simulink model "lab_readyAWU"  (R2020b)
settings: Solver=ode4  StartTime=0.0  StopTime=5  FixedStep=0.001  RelTol=1e-3
values from neighbouring files (symbols this model uses):
  degs2rpm = 0.166666666667    [DIGIT1-BE10.mat]    (also in DIGIT1-FE10.mat; DIGIT1-FE20.mat; DIGIT1-FE4.mat; DIGIT1-TR10.mat)
  filt =     [DIGIT1-BE10.mat]    (also in DIGIT1-FE10.mat; DIGIT1-FE20.mat; DIGIT1-FE4.mat; DIGIT1-TR10.mat)
  rpm2rads = 0.10471975512    [DIGIT1-BE10.mat]    (also in DIGIT1-FE10.mat; DIGIT1-FE20.mat; DIGIT1-FE4.mat; DIGIT1-TR10.mat)
  sens =     [DIGIT1-BE10.mat]    (also in DIGIT1-FE10.mat; DIGIT1-FE20.mat; DIGIT1-FE4.mat; DIGIT1-TR10.mat)
undefined symbols (not defined in the file or in its folder): National_Instruments, PCI
libraries: sldrtlib x3, simulink x1
settings Model: ExtModeTrigDuration=50001  Creator=verrimarco  LastModifiedBy=verrimarco
settings DataIOCC: SaveFormat=StructureWithTime  InspectSignalLogs=on  ReturnWorkspaceOutputs=off  LoggingFileName=out.mat2
settings RTWCC: Description=Simulink Desktop Real-Time  SystemTargetFile=sldrt.tlc  TemplateMakefile=sldrt.tmf  RTWCompilerOptimization=on
settings CodeAppCC: MaxIdLength=95
settings SimulinkDesktopRealTimeCC: TargetPreCompLibLocation=C:\Program Files\MATLAB\R2020b\toolbox\sldrt\lib\win64

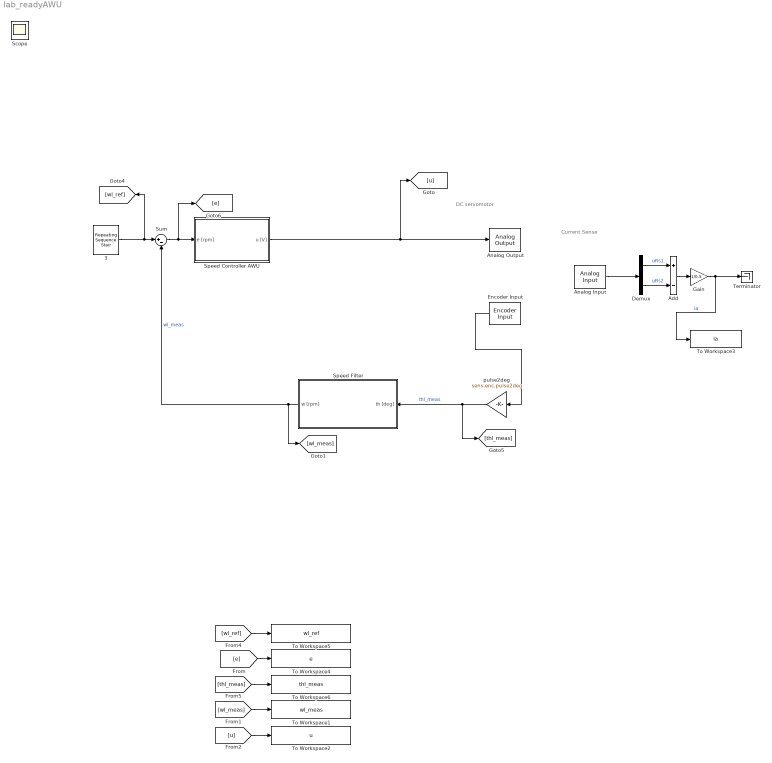
== system lab_readyAWU ==
  note: DC servomotor
  note: Current Sense
  3 : simulink/Sources/Repeating Sequence Stair  OutValues=[450 -450].'  tsamp=3  OutMin=[]  OutMax=[]  OutDataTypeStr=double  OutputDataTypeScalingMode=double  OutDataType=fixdt(0,8)  ConRadixGroup=Best Precision: Vector-wise  OutScaling=2^-12
  Add : Sum  Inputs=+-
  Analog Input : sldrtlib/Analog Input  SampleTime=-1  MaxMissedTicks=10  ShowMissedTicks=off  YieldWhenWaiting=off  DrvName=National_Instruments/PCI-6221  DrvAddress=4294967295  DrvOptions=[0 0 0 2 0]  Channels=[1,2]  RangeMode=1  VoltRange=1  DataType=1
      settings: AttributesFormatString=National Instruments\nPCI-6221 [auto]
  Analog Output : sldrtlib/Analog Output  SampleTime=-1  MaxMissedTicks=10  ShowMissedTicks=off  YieldWhenWaiting=off  DrvName=National_Instruments/PCI-6221  DrvAddress=4294967295  DrvOptions=[0 0 0 2 0]  Channels=1  RangeMode=1  VoltRange=1  InitialValue=0  FinalValue=0
      settings: AttributesFormatString=National Instruments\nPCI-6221 [auto]
  Demux : Demux  Outputs=2
  Encoder Input : sldrtlib/Encoder Input  SampleTime=-1  MaxMissedTicks=10  ShowMissedTicks=off  YieldWhenWaiting=on  DrvName=National_Instruments/PCI-6221  DrvAddress=4294967295  DrvOptions=[0 0 0 2 0]  Channels=1  QuadMode=3  IndexPulse=1  InputFilter=Inf  DataType=1
      settings: AttributesFormatString=National Instruments\nPCI-6221 [auto]
  Gain : Gain  Gain=1/0.5
  Speed Controller AWU : Subsystem
  Speed Filter : Subsystem
  Sum : Sum  Inputs=|+-
  Terminator : Terminator
  To Workspace1 : ToWorkspace  VariableName=wl_meas  SaveFormat=Structure With Time  SampleTime=-1
      settings: Save2DSignal=2-D array (concatenate along first dimension)
  To Workspace2 : ToWorkspace  VariableName=u  SaveFormat=Structure With Time  SampleTime=-1
      settings: Save2DSignal=2-D array (concatenate along first dimension)
  To Workspace3 : ToWorkspace  VariableName=ia  SaveFormat=Structure With Time  SampleTime=-1
  To Workspace4 : ToWorkspace  VariableName=e  SaveFormat=Structure With Time  SampleTime=-1
      settings: Save2DSignal=2-D array (concatenate along first dimension)
  To Workspace5 : ToWorkspace  VariableName=wl_ref  SaveFormat=Structure With Time  SampleTime=-1
      settings: Save2DSignal=2-D array (concatenate along first dimension)
  To Workspace6 : ToWorkspace  VariableName=thl_meas  SaveFormat=Structure With Time  SampleTime=-1
      settings: Save2DSignal=2-D array (concatenate along first dimension)
  pulse2deg : Gain  Gain=sens.enc.pulse2deg
  Scope : Scope
  wires:
  Analog Input/1 -> Demux/1
  Demux/1 -> Add/1  "uRs1"
  Demux/2 -> Add/2  "uRs2"
  Add/1 -> Gain/1
  Gain/1 -> To Workspace3/1, Terminator/1  "ia"
  Speed Controller AWU/1(u [V]) -> [u], Analog Output/1
  pulse2deg/1 -> [thl_meas], Speed Filter/1(th [deg])  "thl_meas"
  Encoder Input/1 -> pulse2deg/1
  [wl_ref] -> To Workspace5/1
  [wl_meas] -> To Workspace1/1
  [u] -> To Workspace2/1
  [thl_meas] -> To Workspace6/1
  Sum/1 -> [e], Speed Controller AWU/1(e [rpm])
  3/1 -> [wl_ref], Sum/1
  Speed Filter/1(w [rpm]) -> Sum/2, [wl_meas]  "wl_meas"
  [e] -> To Workspace4/1

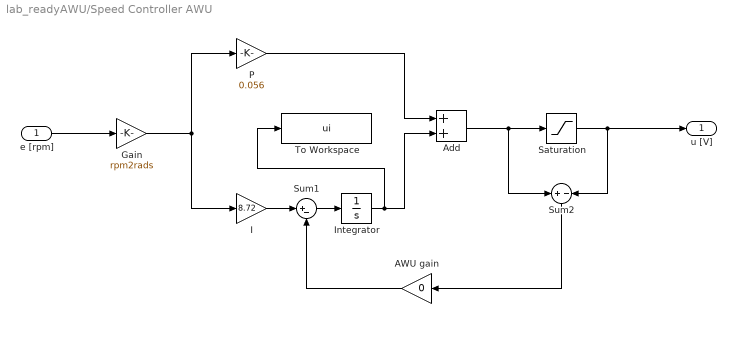
== system lab_readyAWU/Speed Controller AWU ==
  e [rpm] : Inport
  AWU gain : Gain  Gain=0
  Add : Sum
  Gain : Gain  Gain=rpm2rads
  I : Gain  Gain=8.72
  Integrator : Integrator
  P : Gain  Gain=0.056
  Saturation : Saturate  UpperLimit=10  LowerLimit=-10
  Sum1 : Sum  Inputs=|+-
  Sum2 : Sum  Inputs=+-
  To Workspace : ToWorkspace  VariableName=ui  SaveFormat=Structure With Time  SampleTime=-1
  u [V] : Outport
  wires:
  e [rpm]/1 -> Gain/1
  P/1 -> Add/1
  Integrator/1 -> To Workspace/1, Add/2
  Add/1 -> Sum2/1, Saturation/1
  Saturation/1 -> Sum2/2, u [V]/1
  Gain/1 -> I/1, P/1
  Sum1/1 -> Integrator/1
  I/1 -> Sum1/1
  Sum2/1 -> AWU gain/1
  AWU gain/1 -> Sum1/2

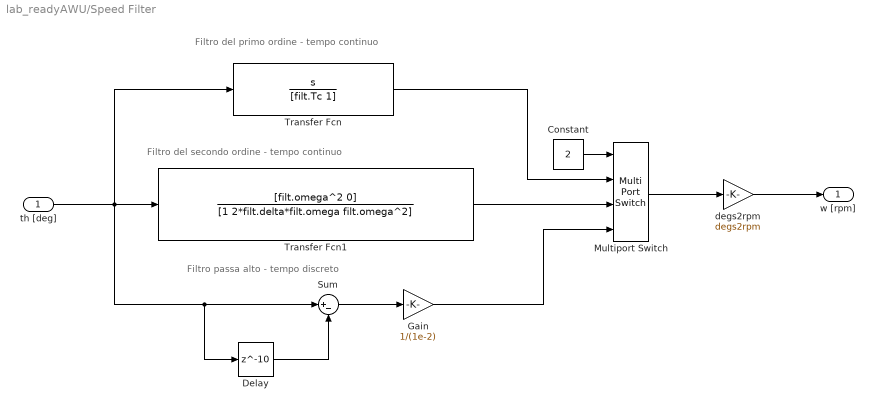
== system lab_readyAWU/Speed Filter ==
  note: Filtro passa alto - tempo discreto
  note: Filtro del secondo ordine - tempo continuo
  note: Filtro del primo ordine - tempo continuo
  th [deg] : Inport
  Constant : Constant  Value=2
  Delay : Delay  DelayLength=10  InitialCondition=0
  Gain : Gain  Gain=1/(1e-2)
  Multiport Switch : MultiPortSwitch
  Sum : Sum  Inputs=|+-
  Transfer Fcn : TransferFcn  Numerator=[1 0]  Denominator=[filt.Tc 1]
  Transfer Fcn1 : TransferFcn  Numerator=[filt.omega^2 0]  Denominator=[1 2*filt.delta*filt.omega filt.omega^2]
  degs2rpm : Gain  Gain=degs2rpm
  w [rpm] : Outport
  wires:
  degs2rpm/1 -> w [rpm]/1
  Transfer Fcn1/1 -> Multiport Switch/3
  Multiport Switch/1 -> degs2rpm/1
  Gain/1 -> Multiport Switch/4
  Delay/1 -> Sum/2
  Sum/1 -> Gain/1
  Constant/1 -> Multiport Switch/1
  Transfer Fcn/1 -> Multiport Switch/2
  th [deg]/1 -> Delay/1, Sum/1, Transfer Fcn/1, Transfer Fcn1/1
